simulink library "orbit"  (R2021b)
settings: Solver=VariableStepAuto  StartTime=0.0  StopTime=10.0  RelTol=1e-3
undefined symbols (not defined in the file or in its folder): J2, mu, R0, Re, V0
libraries: my_math_ops x2, vrlib x1
settings Model: Creator=Davide  LastModifiedBy=Davide

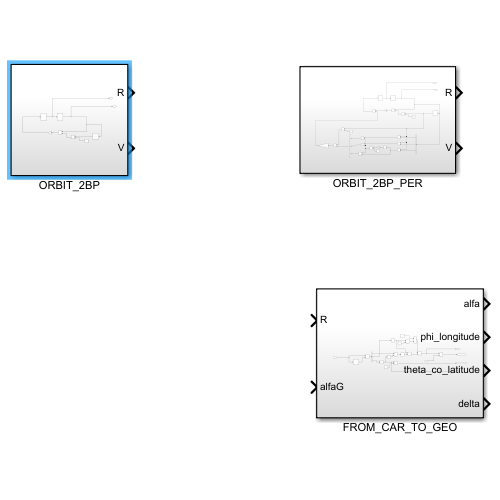
[thumbnail: Simulink's stored preview of the top-level diagram]
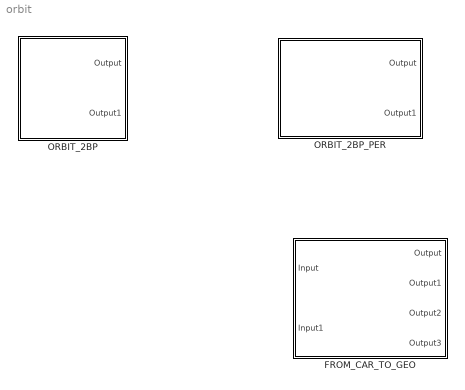
== system orbit ==
  FROM_CAR_TO_GEO : Subsystem
  ORBIT_2BP : Subsystem
  ORBIT_2BP_PER : Subsystem

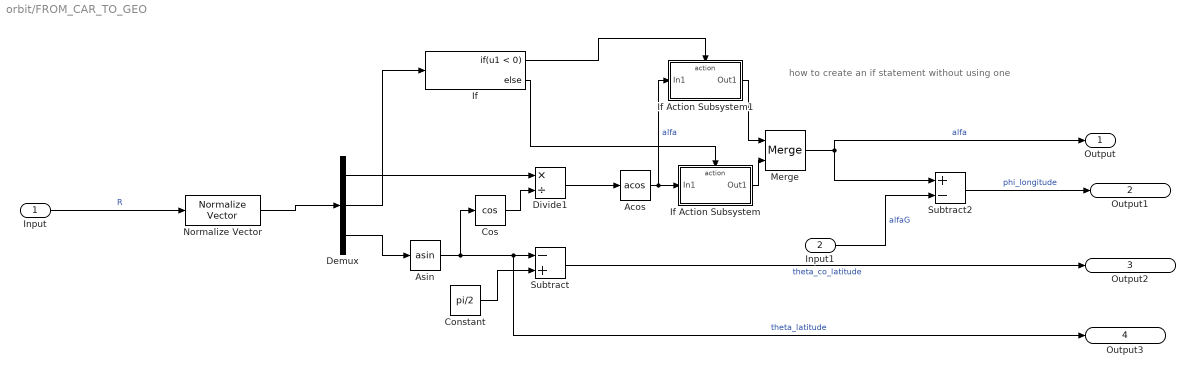
== system orbit/FROM_CAR_TO_GEO ==
  note: how to create an if statement without using one
  Input : Inport
  Input1 : Inport  Port=2
  Acos : Trigonometry  Operator=acos
  Asin : Trigonometry  Operator=asin
  Constant : Constant  Value=pi/2
  Cos : Trigonometry  Operator=cos
  Demux : Demux  Outputs=3
  Divide1 : Product  Inputs=*/
  If : If  IfExpression=u1 < 0
  If Action Subsystem : Subsystem  TreatAsAtomicUnit=on
  If Action Subsystem1 : Subsystem  TreatAsAtomicUnit=on
  Merge : Merge
  Normalize Vector : vrlib/Utilities/Normalize Vector  maxzero=0
  Subtract : Sum  Inputs=-+
  Subtract2 : Sum  Inputs=+-
  Output : Outport
  Output1 : Outport  Port=2
  Output2 : Outport  Port=3
  Output3 : Outport  Port=4
  wires:
  Constant/1 -> Subtract/2
  Asin/1 -> Cos/1, Output3/1, Subtract/1  "theta_latitude"
  Demux/1 -> Divide1/1
  Input/1 -> Normalize Vector/1  "R"
  Input1/1 -> Subtract2/2  "alfaG"
  Cos/1 -> Divide1/2
  Normalize Vector/1 -> Demux/1
  Divide1/1 -> Acos/1
  Demux/3 -> Asin/1
  Subtract/1 -> Output2/1  "theta_co_latitude"
  Subtract2/1 -> Output1/1  "phi_longitude"
  Demux/2 -> If/1
  Merge/1 -> Subtract2/1, Output/1  "alfa"
  Acos/1 -> If Action Subsystem1/1(In1), If Action Subsystem/1(In1)  "alfa"
  If Action Subsystem/1(Out1) -> Merge/2
  If/2 -> If Action Subsystem/Action
  If Action Subsystem1/1(Out1) -> Merge/1
  If/1 -> If Action Subsystem1/Action

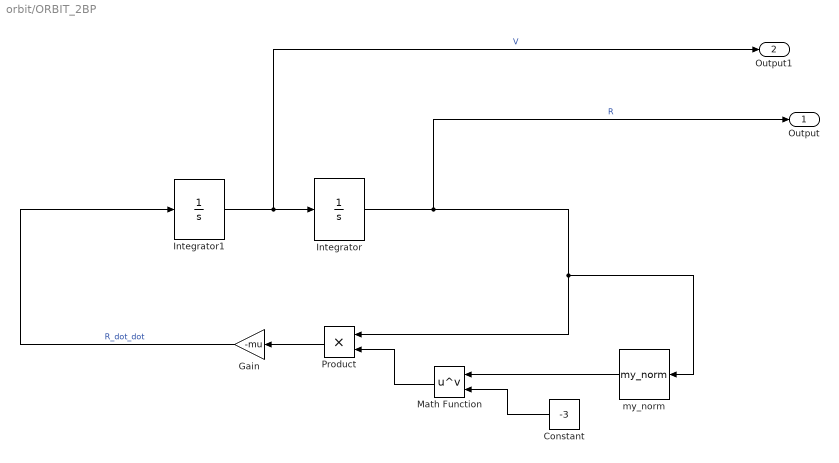
== system orbit/ORBIT_2BP ==
  Constant : Constant  Value=-3
  Gain : Gain  Gain=-mu
  Integrator : Integrator  InitialCondition=R0
  Integrator1 : Integrator  InitialCondition=V0
  Math Function : Math  Operator=pow  SaturateOnIntegerOverflow=on
  Product : Product
  my_norm : my_math_ops/my_norm  SystemSampleTime=-1  VariantActivationTime=update diagram  Latency=0  AutoFrameSizeCalculation=off
  Output : Outport
  Output1 : Outport  Port=2
  wires:
  Constant/1 -> Math Function/2
  Integrator/1 -> Output/1, Product/1, my_norm/1  "R"
  Gain/1 -> Integrator1/1  "R_dot_dot"
  my_norm/1 -> Math Function/1
  Math Function/1 -> Product/2
  Product/1 -> Gain/1
  Integrator1/1 -> Output1/1, Integrator/1  "V"

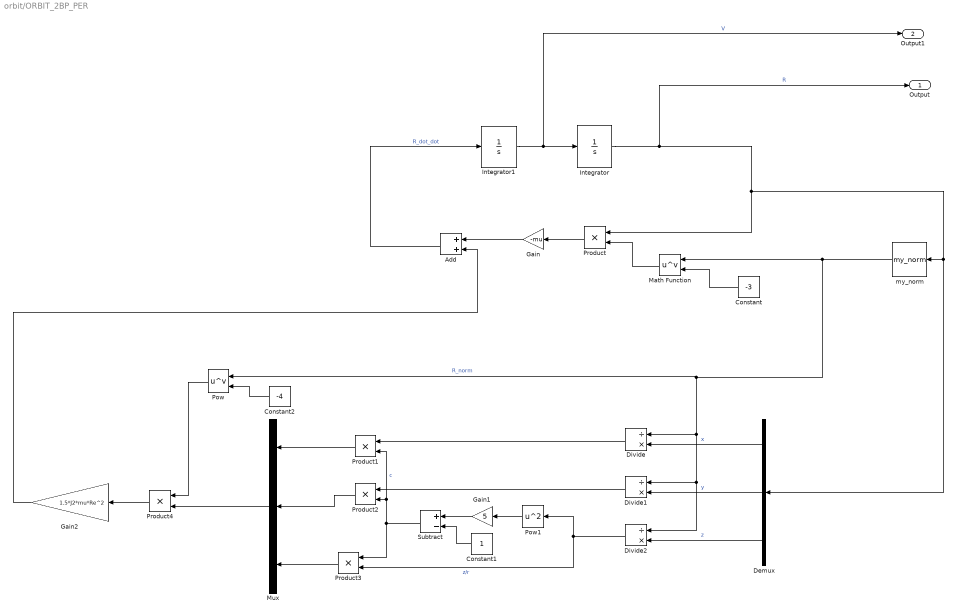
== system orbit/ORBIT_2BP_PER ==
  Add : Sum
  Constant : Constant  Value=-3
  Constant1 : Constant
  Constant2 : Constant  Value=-4
  Demux : Demux  Outputs=3
  Divide : Product  Inputs=/*
  Divide1 : Product  Inputs=/*
  Divide2 : Product  Inputs=/*
  Gain : Gain  Gain=-mu
  Gain1 : Gain  Gain=5
  Gain2 : Gain  Gain=1.5*J2*mu*Re^2
  Integrator : Integrator  InitialCondition=R0
  Integrator1 : Integrator
  Math Function : Math  Operator=pow  SaturateOnIntegerOverflow=on
  Mux : Mux  Inputs=3
  Pow : Math  Operator=pow  RndMeth=Zero  SaturateOnIntegerOverflow=on
  Pow1 : Math  Operator=square  SignedPower=on  RndMeth=Zero  SaturateOnIntegerOverflow=on
  Product{,1..4} (5 alike) : Product
  Subtract : Sum  Inputs=+-
  my_norm : my_math_ops/my_norm  SystemSampleTime=-1  VariantActivationTime=update diagram  Latency=0  AutoFrameSizeCalculation=off
  Output : Outport
  Output1 : Outport  Port=2
  wires:
  Divide2/1 -> Product3/2, Pow1/1  "z/r"
  Subtract/1 -> Product3/1, Product1/2, Product2/2  "c"
  Mux/1 -> Product4/2
  my_norm/1 -> Pow/1, Divide2/1, Divide1/1, Divide/1, Math Function/1  "R_norm"
  Gain1/1 -> Subtract/1
  Integrator1/1 -> Output1/1, Integrator/1  "V"
  Constant/1 -> Math Function/2
  Divide/1 -> Product1/1
  Product4/1 -> Gain2/1
  Integrator/1 -> Output/1, Product/1, Demux/1, my_norm/1  "R"
  Product/1 -> Gain/1
  Math Function/1 -> Product/2
  Product1/1 -> Mux/1
  Demux/1 -> Divide/2  "x"
  Constant2/1 -> Pow/2
  Constant1/1 -> Subtract/2
  Demux/3 -> Divide2/2  "z"
  Pow1/1 -> Gain1/1
  Add/1 -> Integrator1/1  "R_dot_dot"
  Gain/1 -> Add/1
  Product3/1 -> Mux/3
  Product2/1 -> Mux/2
  Gain2/1 -> Add/2
  Demux/2 -> Divide1/2  "y"
  Divide1/1 -> Product2/1
  Pow/1 -> Product4/1

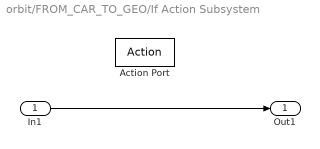
== system orbit/FROM_CAR_TO_GEO/If Action Subsystem ==
  In1 : Inport
  Action Port : ActionPort  ActionPortLabel=else
  Out1 : Outport
  wires:
  In1/1 -> Out1/1

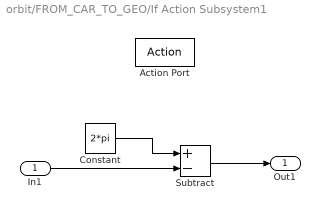
== system orbit/FROM_CAR_TO_GEO/If Action Subsystem1 ==
  In1 : Inport
  Action Port : ActionPort  ActionPortLabel=if(u1 < 0)
  Constant : Constant  Value=2*pi
  Subtract : Sum  Inputs=+-
  Out1 : Outport
  wires:
  In1/1 -> Subtract/2
  Constant/1 -> Subtract/1
  Subtract/1 -> Out1/1
